simulink model "V6___LQR_Regelung"  (R2016a)
settings: Solver=FixedStepDiscrete  StartTime=0.0  StopTime=inf  FixedStep=0.02  RelTol=1e-3
InitFcn:
  | initCallback_lqr_hw
undefined symbols (not defined in the file): Kd
libraries: simulink x1
settings Model: SimulationMode=external  ExtModeLogAll=off  Creator=ich  LastModifiedBy=ich
settings OptimizationCC: OptimizeModelRefInitCode=on  LifeSpan=Inf  MaxStackSize=64
settings HardwareCC: ProdBitPerPointer=32  ProdLargestAtomicInteger=Long  ProdLargestAtomicFloat=Double  ProdWordSize=32  ProdHWDeviceType=ARM Compatible->ARM Cortex
settings RTWCC: SystemTargetFile=ert.tlc  HardwareBoard=STM32F4-Discovery  TemplateMakefile=ert_default_tmf  GenerateReport=on  Toolchain=GNU Tools for ARM Embedded Processors  IncludeHyperlinkInReport=on  LaunchReport=on  GenerateTraceInfo=on  GenerateTraceReport=on  GenerateTraceReportSl=on  GenerateTraceReportSf=on  GenerateTraceReportEml=on
settings RTWCC: CustomInclude=|
  | MotorBlock/include
  | MPU6050/include
settings RTWCC: CustomSource=|
  | MotorBlock/source/ADC.c
  | MotorBlock/source/MotorControl.c
  | MotorBlock/source/stm32f4xx_adc.c
  | MotorBlock/source/stm32f4xx_tim.c
  | MPU6050/source/stm32f4xx_i2c.c
  | MPU6050/source/MPU6050.c
settings CodeAppCC: ForceParamTrailComments=on  IgnoreCustomStorageClasses=off  OperatorAnnotations=on  SimulinkDataObjDesc=on  SFDataObjDesc=on  MATLABFcnDesc=on  InsertBlockDesc=on  MATLABSourceComments=on

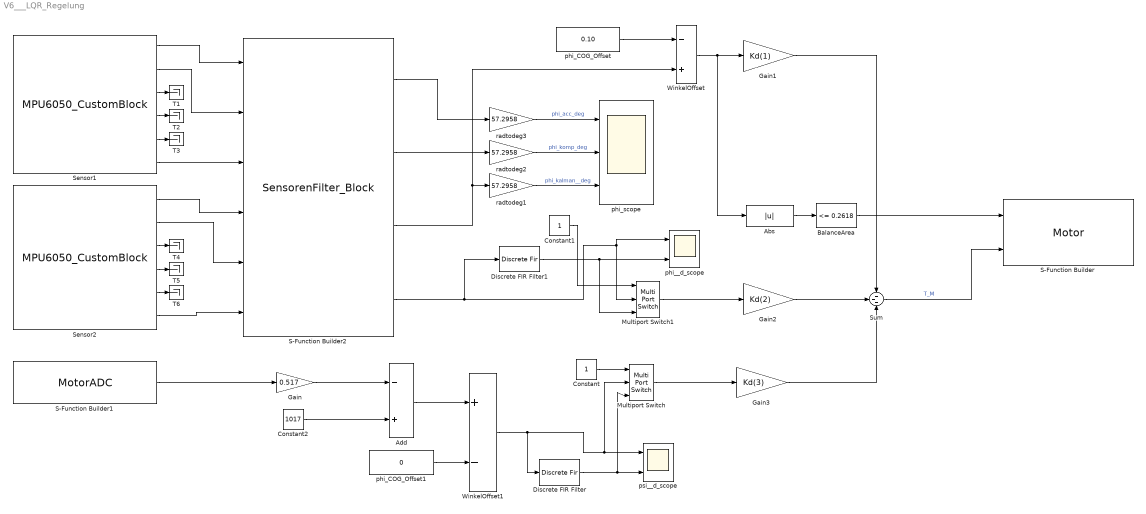
== system V6___LQR_Regelung ==
  Abs : Abs
  Add : Sum  Inputs=-+
  BalanceArea : simulink/Logic and Bit Operations/Compare To Constant  relop=<=  const=0.2618  OutDataTypeStr=boolean
  Constant : Constant
  Constant1 : Constant
  Constant2 : Constant  Value=1017
  Discrete FIR Filter : DiscreteFir  Coefficients=[0.25 0.25 0.25 0.25]
  Discrete FIR Filter1 : DiscreteFir  Coefficients=[0.25 0.25 0.25 0.25]
  Gain : Gain  Gain=0.517
  Gain1 : Gain  Gain=Kd(1)  OutDataTypeStr=Inherit: Inherit via back propagation
  Gain2 : Gain  Gain=Kd(2)  OutDataTypeStr=Inherit: Inherit via back propagation
  Gain3 : Gain  Gain=Kd(3)  OutDataTypeStr=Inherit: Inherit via back propagation
  Multiport Switch : MultiPortSwitch  Inputs=2
  Multiport Switch1 : MultiPortSwitch  Inputs=2
  S-Function Builder : S-Function  InitFcn=try, set_param(gcb,'FunctionName','Motor'), end  FunctionName=Motor  SFunctionModules=Motor_wrapper  SFunctionDeploymentMode=off  EnableBusSupport=off  mask(S-Function Builder){}
      mask help: Simulink:masks:SFunctionBuilder_MD
      mask init:
      | val = [[.9  0.75 0.75 1 1 .9 .9 1]',[1 1 0.75 0.75 .9 .9 1 .9]'];try , sys = get_param(gcb,'SfunBuilderFcnName');if isempty(sys), sys = get_param(gcb,'FunctionName'); end,catch, sys = get_param(gcb,'FunctionName'); end
      settings: CopyFcn=set_param(gcbh,'LinkStatus','none')  PreSaveFcn=try, set_param(gcb,'FunctionName','Motor'), end  OpenFcn=sfunctionwizard(gcbh)
      mask Display: plot(val(:,1),val(:,2)),disp(sys), port_label('input',1,'EnableState'), port_label('input',2,'Torque')
  S-Function Builder1 : S-Function  InitFcn=try, set_param(gcb,'FunctionName','MotorADC'), end  FunctionName=MotorADC  SFunctionModules=MotorADC_wrapper  SFunctionDeploymentMode=off  EnableBusSupport=off  mask(S-Function Builder){}
      mask help: Simulink:masks:SFunctionBuilder_MD
      mask init: same as V6___LQR_Regelung/S-Function Builder
      settings: CopyFcn=set_param(gcbh,'LinkStatus','none')  PreSaveFcn=try, set_param(gcb,'FunctionName','MotorADC'), end  OpenFcn=sfunctionwizard(gcbh)
      mask Display: plot(val(:,1),val(:,2)),disp(sys), port_label('output',1,'MotorADC')
  S-Function Builder2 : S-Function  InitFcn=try, set_param(gcb,'FunctionName','SensorenFilter_Block'), end  FunctionName=SensorenFilter_Block  Parameters=single(0.02)  SFunctionModules=SensorenFilter_Block_wrapper  SFunctionDeploymentMode=off  EnableBusSupport=off  mask(S-Function Builder){}
      mask help: Simulink:masks:SFunctionBuilder_MD
      mask init: same as V6___LQR_Regelung/S-Function Builder
      settings: CopyFcn=set_param(gcbh,'LinkStatus','none')  PreSaveFcn=try, set_param(gcb,'FunctionName','SensorenFilter_Block'), end  OpenFcn=sfunctionwizard(gcbh)
      mask Display: plot(val(:,1),val(:,2)),disp(sys), port_label('input',1,'x1__dd'), port_label('input',2,'y1__dd'), port_label('input',3,'phi1__d'), port_label('input',4,'x2__dd'), port_label('input',5,'y2__dd'), port_label('input',6,'phi2__d'), port_label('output',1,'phi__raw'), port_label('output',2,'phi__comp'), port_label('output',3,'phi__kalman'), port_label('output',4,'phi__d')
  Sensor1 : S-Function  InitFcn=try, set_param(gcb,'FunctionName','MPU6050_CustomBlock'), end  FunctionName=MPU6050_CustomBlock  Parameters=boolean(AD0PinLevel),uint32(LowPassBW)  SFunctionModules=MPU6050_CustomBlock_wrapper  SFunctionDeploymentMode=off  EnableBusSupport=off  mask(S-Function Builder){AD0PinLevel=0, LowPassBW=260}
      mask prompts: AD0PinLevel "Logic-Level of AD0 Pin"; LowPassBW "Low-Pass-Bandwidth [Hz]"
      mask help: Simulink:masks:SFunctionBuilder_MD
      mask init: same as V6___LQR_Regelung/S-Function Builder
      settings: CopyFcn=set_param(gcbh,'LinkStatus','none')  PreSaveFcn=try, set_param(gcb,'FunctionName','MPU6050_CustomBlock'), end  OpenFcn=sfunctionwizard(gcbh)
      mask TypeOptions LowPassBW: 260 | 184 | 94 | 44 | 21 | 10 | 5
      mask Display: plot(val(:,1),val(:,2)),disp(sys), port_label('output',1,'XAcceleration'), port_label('output',2,'YAcceleration'), port_label('output',3,'ZAcceleration'), port_label('output',4,'XAngularVelocity'), port_label('output',5,'YAngularVelocity'), port_label('output',6,'ZAngularVelocity')
  Sensor2 : S-Function  InitFcn=try, set_param(gcb,'FunctionName','MPU6050_CustomBlock'), end  FunctionName=MPU6050_CustomBlock  Parameters=boolean(AD0PinLevel),uint32(LowPassBW)  SFunctionModules=MPU6050_CustomBlock_wrapper  SFunctionDeploymentMode=off  EnableBusSupport=off  mask(S-Function Builder){AD0PinLevel=1, LowPassBW=260}
      mask prompts: AD0PinLevel "Logic-Level of AD0 Pin"; LowPassBW "Low-Pass-Bandwidth [Hz]"
      mask help: Simulink:masks:SFunctionBuilder_MD
      mask init: same as V6___LQR_Regelung/S-Function Builder
      settings: CopyFcn=set_param(gcbh,'LinkStatus','none')  PreSaveFcn=try, set_param(gcb,'FunctionName','MPU6050_CustomBlock'), end  OpenFcn=sfunctionwizard(gcbh)
      mask TypeOptions LowPassBW: 260 | 184 | 94 | 44 | 21 | 10 | 5
      mask Display: plot(val(:,1),val(:,2)),disp(sys), port_label('output',1,'XAcceleration'), port_label('output',2,'YAcceleration'), port_label('output',3,'ZAcceleration'), port_label('output',4,'XAngularVelocity'), port_label('output',5,'YAngularVelocity'), port_label('output',6,'ZAngularVelocity')
  Sum : Sum  Inputs=---  OutDataTypeStr=Inherit: Inherit via back propagation
  T{1..6} (6 alike) : Terminator
  WinkelOffset : Sum  Inputs=-+
  WinkelOffset1 : Sum  Inputs=+-
  phi_COG_Offset : Constant  Value=0.10  OutDataTypeStr=Inherit: Inherit via back propagation
  phi_COG_Offset1 : Constant  Value=0  OutDataTypeStr=Inherit: Inherit via back propagation
  phi__d_scope : Scope  NumInputPorts=2
  phi_scope : Scope  NumInputPorts=3
  psi__d_scope : Scope  NumInputPorts=2
  radtodeg1 : Gain  Gain=57.2958
  radtodeg2 : Gain  Gain=57.2958
  radtodeg3 : Gain  Gain=57.2958
  wires:
  BalanceArea/1 -> S-Function Builder/1
  Sum/1 -> S-Function Builder/2  "T_M"
  Constant2/1 -> Add/2
  Gain/1 -> Add/1
  WinkelOffset1/1 -> Discrete FIR Filter/1, Multiport Switch/2, psi__d_scope/1
  S-Function Builder1/1 -> Gain/1
  Sensor1/3 -> T1/1
  Sensor1/4 -> T2/1
  Sensor1/5 -> T3/1
  Sensor2/5 -> T6/1
  Sensor2/4 -> T5/1
  Sensor2/3 -> T4/1
  S-Function Builder2/3 -> WinkelOffset/2, radtodeg1/1
  S-Function Builder2/4 -> Discrete FIR Filter1/1, Multiport Switch1/2, phi__d_scope/1
  radtodeg1/1 -> phi_scope/3  "phi_kalman__deg"
  Gain2/1 -> Sum/2
  Gain1/1 -> Sum/1
  Gain3/1 -> Sum/3
  S-Function Builder2/2 -> radtodeg2/1
  S-Function Builder2/1 -> radtodeg3/1
  WinkelOffset/1 -> Abs/1, Gain1/1
  phi_COG_Offset/1 -> WinkelOffset/1
  Abs/1 -> BalanceArea/1
  Sensor1/1 -> S-Function Builder2/1
  Sensor1/2 -> S-Function Builder2/2
  Sensor2/6 -> S-Function Builder2/6
  Sensor1/6 -> S-Function Builder2/3
  Sensor2/1 -> S-Function Builder2/4
  Sensor2/2 -> S-Function Builder2/5
  Add/1 -> WinkelOffset1/1
  phi_COG_Offset1/1 -> WinkelOffset1/2
  radtodeg2/1 -> phi_scope/2  "phi_komp_deg"
  radtodeg3/1 -> phi_scope/1  "phi_acc_deg"
  Discrete FIR Filter/1 -> Multiport Switch/3, psi__d_scope/2
  Multiport Switch/1 -> Gain3/1
  Constant/1 -> Multiport Switch/1
  Discrete FIR Filter1/1 -> Multiport Switch1/3, phi__d_scope/2
  Constant1/1 -> Multiport Switch1/1
  Multiport Switch1/1 -> Gain2/1
